simulink model "EKF_03"  (R2015a)
settings: Solver=ode45  StartTime=0.0  StopTime=40  RelTol=1e-3
model workspace: external: MAT-File Init_Model_02_Simulink.mat (data not in the file)
values from neighbouring files (symbols this model uses):
  Cov_nu = [0.005 0 0 0 ... (first row only)    [InitOOSM.m]    (also in InitSIL.m; Init_Model_02_Simulink.m; Init_Model_02_Simulink_SIL1.m)
  Cov_r = [0.003 0 0 ... (first row only)    [InitOOSM.m]    (also in InitSIL.m; Init_Model_02_Simulink.m; Init_Model_02_Simulink_SIL1.m)
  e_force_x = 0    [InitOOSM.m]    (also in InitSIL.m; Init_Model_02_Simulink.m; Init_Model_02_Simulink_SIL1.m)
  e_force_y = 0    [InitOOSM.m]    (also in InitSIL.m; Init_Model_02_Simulink.m; Init_Model_02_Simulink_SIL1.m)
  e_force_z = 0    [InitOOSM.m]    (also in InitSIL.m; Init_Model_02_Simulink.m; Init_Model_02_Simulink_SIL1.m)
  ita = [0.5;0.5;0.5;0.5]    [InitOOSM.m]    (also in InitSIL.m; Init_Model_02_Simulink.m = [0.12; 0.05; -0.15; 0.98]; Init_Model_02_Simulink_SIL1.m)
  n = 0.00    (= 0)    [InitOOSM.m]    (also in InitSIL.m; Init_Model_02_Simulink.m = 0.0012; Init_Model_02_Simulink_SIL1.m)
  P_d = Simulink.Signal    [InitOOSM.m]    (also in InitSIL.m; Init_Model_02_Simulink.m; Init_Model_02_Simulink_SIL1.m)
  P_k = Simulink.Signal    [InitOOSM.m]    (also in InitSIL.m; Init_Model_02_Simulink.m; Init_Model_02_Simulink_SIL1.m)
  p_x = 0.75    [InitOOSM.m]    (also in InitSIL.m; Init_Model_02_Simulink.m; Init_Model_02_Simulink_SIL1.m)
  p_y = 0.125    [InitOOSM.m]    (also in InitSIL.m; Init_Model_02_Simulink.m; Init_Model_02_Simulink_SIL1.m)
  p_z = -0.8    [InitOOSM.m]    (also in InitSIL.m; Init_Model_02_Simulink.m; Init_Model_02_Simulink_SIL1.m)
  parameter_gravitation = 3.986005E+14    (= 398600500000000)    [InitOOSM.m]    (also in InitSIL.m; Init_Model_02_Simulink.m; Init_Model_02_Simulink_SIL1.m)
  rho = [0.04;0;0.3]    [InitOOSM.m]    (also in InitSIL.m; Init_Model_02_Simulink.m = [0.2; 0.1; 0.05]; Init_Model_02_Simulink_SIL1.m)
  rho_c = [-0.00017;   -0.9780;   -0.1854]    [InitOOSM.m]    (also in InitSIL.m = [0.00036;   -0.9865;   -0.1854]; Init_Model_02_Simulink.m = [0; 0; 0.9]; Init_Model_02_Simulink_SIL1.m = [0.00036;   -0.9865;   -0.1854])
  sig_f = 2E-6    (= 2e-06)    [InitOOSM.m]    (also in InitSIL.m; Init_Model_02_Simulink.m; Init_Model_02_Simulink_SIL1.m)
  sig_tau = 2.5E-5    (= 2.5e-05)    [InitOOSM.m]    (also in InitSIL.m; Init_Model_02_Simulink.m; Init_Model_02_Simulink_SIL1.m)
  t_delta = 0.2    [InitOOSM.m]    (also in InitSIL.m; Init_Model_02_Simulink.m = 0.1; Init_Model_02_Simulink_SIL1.m)
  t_Kalman = 0.01    [InitOOSM.m]    (also in InitSIL.m; Init_Model_02_Simulink.m; Init_Model_02_Simulink_SIL1.m)
  t_Sim = 0.001    [InitOOSM.m]    (also in InitSIL.m; Init_Model_02_Simulink.m; Init_Model_02_Simulink_SIL1.m)
  tau_1 = 0    [InitOOSM.m]    (also in InitSIL.m; Init_Model_02_Simulink.m; Init_Model_02_Simulink_SIL1.m)
  tau_2 = 0    [InitOOSM.m]    (also in InitSIL.m; Init_Model_02_Simulink.m; Init_Model_02_Simulink_SIL1.m)
  tau_3 = 0    [InitOOSM.m]    (also in InitSIL.m; Init_Model_02_Simulink.m; Init_Model_02_Simulink_SIL1.m)
  U_n_d = Simulink.Signal    [InitOOSM.m]    (also in InitSIL.m; Init_Model_02_Simulink.m; Init_Model_02_Simulink_SIL1.m)
  X_a_0 = [0; 0; 0; 1; 0; 0; 0; 0; 0; 0; 0; 0; 0;0;0;0;0;0;0;1]    [InitOOSM.m]    (also in InitSIL.m = [0; 0; 0; 1; 0; 0; 0; 0; 0; 0; 0; 0; 0]; Init_Model_02_Simulink.m = [0; 0; 0; 1; 0; 0; 0; 0; 0; 0; 0; 0; 0]; Init_Model_02_Simulink_SIL1.m = [0;0;0.707;0.707;0.2;-0.02;0.0001;0.02;-1.80;0.50;-0.05;0.00)
  x_d = Simulink.Signal    [InitOOSM.m]    (also in InitSIL.m; Init_Model_02_Simulink.m; Init_Model_02_Simulink_SIL1.m)
  x_k = Simulink.Signal    [InitOOSM.m]    (also in InitSIL.m; Init_Model_02_Simulink.m; Init_Model_02_Simulink_SIL1.m)
undefined symbols (not defined in the file or in its folder): des, gcbh
libraries: simulink x5, dspmtrx3 x1
(part 3 of 5)

== system EKF_03/OOSM_KF/OOSM_KF/Initialize OOSM/Create State error covariance (P) ==
  X_a : Inport
  P_previous : Inport  Port=2
  del_t : Inport  Port=3
  Add : Sum
  Math Function : Math  Operator=transpose  SaturateOnIntegerOverflow=on
  Matrix Concatenate : Concatenate  Mode=Multidimensional array  ConcatenateDimension=2
  Matrix Concatenate1 : Concatenate  Mode=Multidimensional array
  Matrix Concatenate2 : Concatenate  Mode=Multidimensional array  ConcatenateDimension=2
  Process noise covariance [rotational] : Subsystem
  Process noise covariance [translational] : Subsystem
  Product : Product  Inputs=3  Multiplication=Matrix(*)
  State Propagation : Subsystem
  zeros(6,6) : Constant  Value=zeros(6,6)
  P_current : Outport
  wires:
  Math Function/1 -> Product/3
  P_previous/1 -> Product/2
  Add/1 -> P_current/1
  X_a/1 -> State Propagation/1("X_a(t)\t")
  Product/1 -> Add/2
  Matrix Concatenate1/1 -> Add/1
  Matrix Concatenate2/1 -> Matrix Concatenate1/2
  Matrix Concatenate/1 -> Matrix Concatenate1/1
  Process noise covariance [translational]/1(Q_t) -> Matrix Concatenate2/2
  zeros(6,6)/1 -> Matrix Concatenate2/1, Matrix Concatenate/2
  Process noise covariance [rotational]/1(Q_r) -> Matrix Concatenate/1
  State Propagation/1(Phi) -> Math Function/1, Product/1, Process noise covariance [rotational]/1(Phi)
  del_t/1 -> State Propagation/2(del_t), Process noise covariance [rotational]/2(del_t), Process noise covariance [translational]/1(del_t)

== system EKF_03/OOSM_KF/OOSM_KF/Initialize OOSM/Propagate_state (full) ==
  X_a(k-n) : Inport
  del_t : Inport  Port=2
  Bus Selector : BusSelector  OutputSignals=omega,r,r_dot
  Create q_nominal : Subsystem  TreatAsAtomicUnit=on
  Data Store Write : DataStoreWrite  DataStoreName=q_nominal_d
  Mux : Mux  Inputs=3
  Mux1 : Mux  Inputs=2
  Product : Product  Multiplication=Matrix(*)
  Selector : Selector  NumberOfDimensions=2  InputPortWidth=3  IndexOptions=Index vector (dialog),Index vector (dialog)  Indices=[4:12],[4:12]  OutputSizes=1,1
  State Propagation1 : Subsystem
  X_a(k-n,d) : Outport
  wires:
  X_a(k-n)/1 -> Bus Selector/1, Create q_nominal/1(X_a), State Propagation1/1("X_a(t)\t")
  Mux1/1 -> X_a(k-n,d)/1
  Bus Selector/1 -> Mux/1  "<omega>"
  Bus Selector/2 -> Mux/2  "<r>"
  Selector/1 -> Product/1
  Mux/1 -> Product/2
  Bus Selector/3 -> Mux/3  "<r_dot>"
  Product/1 -> Mux1/2
  Create q_nominal/1(Out1) -> Data Store Write/1, Mux1/1
  State Propagation1/1(Phi) -> Selector/1
  del_t/1 -> Create q_nominal/2(del_t), State Propagation1/2(del_t)

== system EKF_03/OOSM_KF/OOSM_KF/Initialize OOSM/State Propagation ==
  "X_a(t)\t" : Inport
  del_t : Inport  Port=2
  Create M : Subsystem
  MATLAB Function : MATLAB Function  TreatAsAtomicUnit=on
  n : Constant  Value=n
  p : Constant  Value=[p_x;p_y;p_z]
  Phi : Outport
  wires:
  p/1 -> Create M/2(p), MATLAB Function/4(p)
  n/1 -> MATLAB Function/2(n)
  del_t/1 -> MATLAB Function/3(t_Kalman)
  MATLAB Function/1(Phi) -> Phi/1
  "X_a(t)\t"/1 -> Create M/1("X_a "), MATLAB Function/1(X_a)
  Create M/1(M) -> MATLAB Function/5(M)

== system EKF_03/OOSM_KF/OOSM_KF/State Propagation1/Create M ==
  "X_a " : Inport
  p : Inport  Port=2
  0 : Constant  Value=0
  Bus Selector1 : BusSelector  OutputSignals=omega
  Bus Selector2 : BusSelector  OutputSignals=omega_x,omega_y,omega_z
  Create 3x3 matrix : Subsystem
  Demux : Demux  Outputs=3
  Product{,1..5} (6 alike) : Product
  M : Outport
  wires:
  Demux/1 -> Product1/1, Product/1
  p/1 -> Demux/1
  0/1 -> Create 3x3 matrix/1(a11), Create 3x3 matrix/9(a33), Create 3x3 matrix/5(a22)
  Product4/1 -> Create 3x3 matrix/7(a31)
  Product1/1 -> Create 3x3 matrix/3(a13)
  Bus Selector2/3 -> Product/2, Product2/2  "<omega_z>"
  Product5/1 -> Create 3x3 matrix/8(a32)
  Demux/3 -> Product5/1, Product4/1
  Bus Selector1/1 -> Bus Selector2/1  "<omega>"
  Product2/1 -> Create 3x3 matrix/4(a21)
  Demux/2 -> Product3/1, Product2/1
  Product/1 -> Create 3x3 matrix/2(a12)
  Bus Selector2/2 -> Product1/2, Product4/2  "<omega_y>"
  Create 3x3 matrix/1(Matrix) -> M/1
  Bus Selector2/1 -> Product5/2, Product3/2  "<omega_x>"
  Product3/1 -> Create 3x3 matrix/6(a23)
  "X_a "/1 -> Bus Selector1/1

== system EKF_03/OOSM_KF/Subsystem/Enabled Subsystem/Create H_k ==
  rho : Inport
  q_nominal : Inport  Port=2
  "Create Rotation Matrix " : Subsystem
  Create Skew Symmetric : Subsystem
  Gain : Gain  Gain=-2
  Matrix Concatenate : Concatenate  NumInputs=4  Mode=Multidimensional array  ConcatenateDimension=2
  Matrix Concatenate1 : Concatenate  NumInputs=4  Mode=Multidimensional array  ConcatenateDimension=2
  Matrix Concatenate2 : Concatenate  Mode=Multidimensional array
  Product : Product  Multiplication=Matrix(*)
  eye_3_3 : Constant  Value=eye(3,3)
  zeros_3_3 : Constant  Value=zeros(3,3)
  H_k : Outport
  wires:
  q_nominal/1 -> "Create Rotation Matrix "/1(q)
  Matrix Concatenate2/1 -> H_k/1
  "Create Rotation Matrix "/1(R) -> Product/1
  Product/1 -> Gain/1
  eye_3_3/1 -> Matrix Concatenate1/1, Matrix Concatenate/3
  zeros_3_3/1 -> Matrix Concatenate1/2, Matrix Concatenate1/4, Matrix Concatenate1/3, Matrix Concatenate/4, Matrix Concatenate/2
  Create Skew Symmetric/1(skew symmetric Matrix) -> Product/2
  Gain/1 -> Matrix Concatenate/1
  rho/1 -> Create Skew Symmetric/1(vector)
  Matrix Concatenate1/1 -> Matrix Concatenate2/2
  Matrix Concatenate/1 -> Matrix Concatenate2/1

== system EKF_03/Plant/Dynamic Model (Differential equations)/Orbital Dynamics /Create Skew Symmetric ==
  vector : Inport
  0 : Constant  Value=0
  Create 3x3 matrix : Subsystem
  Demux : Demux  Outputs=3
  Demux1 : Demux  Outputs=3
  Gain : Gain  Gain=-1
  skew symmetric Matrix : Outport
  wires:
  0/1 -> Create 3x3 matrix/1(a11), Create 3x3 matrix/5(a22), Create 3x3 matrix/9(a33)
  Demux/3 -> Create 3x3 matrix/2(a12)
  Demux1/2 -> Create 3x3 matrix/3(a13)
  Demux1/3 -> Create 3x3 matrix/4(a21)
  Demux/1 -> Create 3x3 matrix/6(a23)
  vector/1 -> Demux1/1, Gain/1
  Create 3x3 matrix/1(Matrix) -> skew symmetric Matrix/1
  Gain/1 -> Demux/1
  Demux/2 -> Create 3x3 matrix/7(a31)
  Demux1/1 -> Create 3x3 matrix/8(a32)

== system EKF_03/Plant/Dynamic Model (Differential equations)/Orbital Dynamics /norm  ==
  vector : Inport
  Dot Product : DotProduct  InputSameDT=on  OutDataTypeStr=Inherit: Inherit via internal rule
  Sqrt : Sqrt  SaturateOnIntegerOverflow=on
  "norm " : Outport
  wires:
  Dot Product/1 -> Sqrt/1
  vector/1 -> Dot Product/2, Dot Product/1
  Sqrt/1 -> "norm "/1

== system EKF_03/Plant/Dynamic Model (Differential equations)/Rotational Dynamics/Create  J ==
  p : Inport
  0 : Constant  Value=0
  1 : Constant
  Create 3x3 matrix : Subsystem
  Fcn : Fcn  Expr=1-u(2)/1+u(1)
  Fcn1 : Fcn  Expr=1+u(3)/1-u(1)
  "J_k " : Outport
  wires:
  Fcn/1 -> Create 3x3 matrix/5(a22)
  p/1 -> Fcn1/1, Fcn/1
  0/1 -> Create 3x3 matrix/2(a12), Create 3x3 matrix/3(a13), Create 3x3 matrix/4(a21), Create 3x3 matrix/6(a23), Create 3x3 matrix/7(a31), Create 3x3 matrix/8(a32)
  Create 3x3 matrix/1(Matrix) -> "J_k "/1
  Fcn1/1 -> Create 3x3 matrix/9(a33)
  1/1 -> Create 3x3 matrix/1(a11)

== system EKF_03/Plant/Dynamic Model (Differential equations)/Rotational Dynamics/Create Psi ==
  "omega " : Inport
  p : Inport  Port=2
  Create Psi : Concatenate  NumInputs=3
  Demux : Demux  Outputs=3
  Demux1 : Demux  Outputs=3
  Product{,1..5} (6 alike) : Product
  Psi : Outport
  wires:
  Demux1/3 -> Product1/2, Product3/2
  p/1 -> Demux/1
  Demux/3 -> Product4/1
  Product4/1 -> Create Psi/3
  Demux1/1 -> Product5/2, Product3/1
  Demux1/2 -> Product1/1, Product5/1
  Product2/1 -> Create Psi/2
  Demux/1 -> Product/1
  Create Psi/1 -> Psi/1
  Demux/2 -> Product2/1
  Product/1 -> Create Psi/1
  Product1/1 -> Product/2
  Product5/1 -> Product4/2
  Product3/1 -> Product2/2
  "omega "/1 -> Demux1/1

== system EKF_03/Plots and display/Create Measurements [Pose]1/Create Measurements [Position]/Create Rotation Matrix  ==
  q : Inport
  Add : Sum
  Add5 : Sum  Inputs=+++
  Constant1 : Constant  Value=-1
  Create Skew Symmetric : Subsystem
  Gain : Gain  Gain=2
  Gain1 : Gain  Gain=2
  Gain2 : Gain  Gain=2
  I : Constant  Value=eye(3,3)
  Math Function : Math  Operator=square  SaturateOnIntegerOverflow=on
  Math Function1 : Math  Operator=transpose  SaturateOnIntegerOverflow=on
  Product1 : Product
  Product2 : Product
  Product3 : Product  Multiplication=Matrix(*)
  Selector2 : Selector  NumberOfDimensions=2  InputPortWidth=3  IndexOptions=Index vector (dialog),Index vector (dialog)  Indices=[1 2 3],1  OutputSizes=1,1
  Selector3 : Selector  NumberOfDimensions=2  InputPortWidth=3  IndexOptions=Index vector (dialog),Index vector (dialog)  Indices=[4],1  OutputSizes=1,1
  R : Outport
  wires:
  q/1 -> Selector2/1, Selector3/1
  Add5/1 -> R/1
  Product3/1 -> Gain2/1
  Math Function1/1 -> Product3/2
  Product1/1 -> Add5/3
  Gain1/1 -> Product2/1
  Create Skew Symmetric/1(skew symmetric Matrix) -> Gain1/1
  Product2/1 -> Add5/2
  Gain2/1 -> Add5/1
  Selector2/1 -> Create Skew Symmetric/1(vector), Product3/1, Math Function1/1
  I/1 -> Product1/2
  Add/1 -> Product1/1
  Selector3/1 -> Math Function/1, Product2/2
  Constant1/1 -> Add/2
  Math Function/1 -> Gain/1
  Gain/1 -> Add/1

== system EKF_03/Create synthetic measurements [Pose]/Create Measurements [Position]/Create Rotation Matrix /Create Skew Symmetric/Create 3x3 matrix ==
  a11 : Inport
  a12 : Inport  Port=2
  a13 : Inport  Port=3
  a21 : Inport  Port=4
  a22 : Inport  Port=5
  a23 : Inport  Port=6
  a31 : Inport  Port=7
  a32 : Inport  Port=8
  a33 : Inport  Port=9
  Math Function : Math  Operator=transpose  SaturateOnIntegerOverflow=on
  Reshape (9) to [3x3] column-major : Reshape  OutputDimensionality=Customize  OutputDimensions=[3,3]
  Vector Concatenate : Concatenate  NumInputs=9
  Matrix : Outport
  wires:
  a33/1 -> Vector Concatenate/9
  a22/1 -> Vector Concatenate/5
  Vector Concatenate/1 -> Reshape (9) to [3x3] column-major/1
  a11/1 -> Vector Concatenate/1
  a12/1 -> Vector Concatenate/2
  a13/1 -> Vector Concatenate/3
  a23/1 -> Vector Concatenate/6
  a31/1 -> Vector Concatenate/7
  a32/1 -> Vector Concatenate/8
  a21/1 -> Vector Concatenate/4
  Reshape (9) to [3x3] column-major/1 -> Math Function/1
  Math Function/1 -> Matrix/1

== system EKF_03/EKF/Measurement Update/Compute_K_d/Create H_k/Create Rotation Matrix  ==
  q : Inport
  Add : Sum
  Add5 : Sum  Inputs=+++
  Constant1 : Constant  Value=-1
  Create Skew Symmetric : Subsystem
  Gain : Gain  Gain=2
  Gain1 : Gain  Gain=2
  Gain2 : Gain  Gain=2
  I : Constant  Value=eye(3,3)
  Math Function : Math  Operator=square  SaturateOnIntegerOverflow=on
  Math Function1 : Math  Operator=transpose  SaturateOnIntegerOverflow=on
  Product1 : Product
  Product2 : Product
  Product3 : Product  Multiplication=Matrix(*)
  Selector2 : Selector  NumberOfDimensions=2  InputPortWidth=3  IndexOptions=Index vector (dialog),Index vector (dialog)  Indices=[1 2 3],1  OutputSizes=1,1
  Selector3 : Selector  NumberOfDimensions=2  InputPortWidth=3  IndexOptions=Index vector (dialog),Index vector (dialog)  Indices=[4],1  OutputSizes=1,1
  R : Outport
  wires:
  Gain/1 -> Add/1
  Math Function/1 -> Gain/1
  Constant1/1 -> Add/2
  Selector3/1 -> Product2/2, Math Function/1
  Add/1 -> Product1/1
  I/1 -> Product1/2
  Selector2/1 -> Math Function1/1, Product3/1, Create Skew Symmetric/1(vector)
  Gain2/1 -> Add5/1
  Product2/1 -> Add5/2
  Create Skew Symmetric/1(skew symmetric Matrix) -> Gain1/1
  Gain1/1 -> Product2/1
  Product1/1 -> Add5/3
  Math Function1/1 -> Product3/2
  Product3/1 -> Gain2/1
  Add5/1 -> R/1
  q/1 -> Selector3/1, Selector2/1

== system EKF_03/EKF/Measurement Update/Compute_K_d/Create H_k/Create Skew Symmetric ==
  vector : Inport
  0 : Constant  Value=0
  Create 3x3 matrix : Subsystem
  Demux : Demux  Outputs=3
  Demux1 : Demux  Outputs=3
  Gain : Gain  Gain=-1
  skew symmetric Matrix : Outport
  wires:
  0/1 -> Create 3x3 matrix/1(a11), Create 3x3 matrix/9(a33), Create 3x3 matrix/5(a22)
  Demux/3 -> Create 3x3 matrix/2(a12)
  Demux1/2 -> Create 3x3 matrix/3(a13)
  Demux1/3 -> Create 3x3 matrix/4(a21)
  Demux/1 -> Create 3x3 matrix/6(a23)
  vector/1 -> Demux1/1, Gain/1
  Create 3x3 matrix/1(Matrix) -> skew symmetric Matrix/1
  Gain/1 -> Demux/1
  Demux/2 -> Create 3x3 matrix/7(a31)
  Demux1/1 -> Create 3x3 matrix/8(a32)

== system EKF_03/EKF/Measurement Update/Create H_k/Create Rotation Matrix /Create Skew Symmetric ==
  vector : Inport
  0 : Constant  Value=0
  Create 3x3 matrix : Subsystem
  Demux : Demux  Outputs=3
  Demux1 : Demux  Outputs=3
  Gain : Gain  Gain=-1
  skew symmetric Matrix : Outport
  wires:
  0/1 -> Create 3x3 matrix/1(a11), Create 3x3 matrix/9(a33), Create 3x3 matrix/5(a22)
  Demux/3 -> Create 3x3 matrix/2(a12)
  Demux1/2 -> Create 3x3 matrix/3(a13)
  Demux1/3 -> Create 3x3 matrix/4(a21)
  Demux/1 -> Create 3x3 matrix/6(a23)
  vector/1 -> Demux1/1, Gain/1
  Create 3x3 matrix/1(Matrix) -> skew symmetric Matrix/1
  Gain/1 -> Demux/1
  Demux/2 -> Create 3x3 matrix/7(a31)
  Demux1/1 -> Create 3x3 matrix/8(a32)

== system EKF_03/EKF/Measurement Update/Create H_k/Create Skew Symmetric/Create 3x3 matrix ==
  a11 : Inport
  a12 : Inport  Port=2
  a13 : Inport  Port=3
  a21 : Inport  Port=4
  a22 : Inport  Port=5
  a23 : Inport  Port=6
  a31 : Inport  Port=7
  a32 : Inport  Port=8
  a33 : Inport  Port=9
  Math Function : Math  Operator=transpose  SaturateOnIntegerOverflow=on
  Reshape (9) to [3x3] column-major : Reshape  OutputDimensionality=Customize  OutputDimensions=[3,3]
  Vector Concatenate : Concatenate  NumInputs=9
  Matrix : Outport
  wires:
  a33/1 -> Vector Concatenate/9
  a22/1 -> Vector Concatenate/5
  Vector Concatenate/1 -> Reshape (9) to [3x3] column-major/1
  a11/1 -> Vector Concatenate/1
  a12/1 -> Vector Concatenate/2
  a13/1 -> Vector Concatenate/3
  a23/1 -> Vector Concatenate/6
  a31/1 -> Vector Concatenate/7
  a32/1 -> Vector Concatenate/8
  a21/1 -> Vector Concatenate/4
  Reshape (9) to [3x3] column-major/1 -> Math Function/1
  Math Function/1 -> Matrix/1

== system EKF_03/EKF/Measurement Update/Create X_a from X/Create q_nominal /norm  ==
  vector : Inport
  Dot Product : DotProduct  InputSameDT=on  OutDataTypeStr=Inherit: Inherit via internal rule
  "norm " : Outport
  wires:
  vector/1 -> Dot Product/2, Dot Product/1
  Dot Product/1 -> "norm "/1

== system EKF_03/EKF/Measurement Update/Create h/Create Rotation Matrix /Create Skew Symmetric ==
  vector : Inport
  0 : Constant  Value=0
  Create 3x3 matrix : Subsystem
  Demux : Demux  Outputs=3
  Demux1 : Demux  Outputs=3
  Gain : Gain  Gain=-1
  skew symmetric Matrix : Outport
  wires:
  0/1 -> Create 3x3 matrix/1(a11), Create 3x3 matrix/9(a33), Create 3x3 matrix/5(a22)
  Demux/3 -> Create 3x3 matrix/2(a12)
  Demux1/2 -> Create 3x3 matrix/3(a13)
  Demux1/3 -> Create 3x3 matrix/4(a21)
  Demux/1 -> Create 3x3 matrix/6(a23)
  vector/1 -> Demux1/1, Gain/1
  Create 3x3 matrix/1(Matrix) -> skew symmetric Matrix/1
  Gain/1 -> Demux/1
  Demux/2 -> Create 3x3 matrix/7(a31)
  Demux1/1 -> Create 3x3 matrix/8(a32)

== system EKF_03/EKF/Measurement Update/Create h/Subsystem/norm  ==
  vector : Inport
  Dot Product : DotProduct  InputSameDT=on  OutDataTypeStr=Inherit: Inherit via internal rule
  "norm " : Outport
  wires:
  vector/1 -> Dot Product/2, Dot Product/1
  Dot Product/1 -> "norm "/1

== system EKF_03/EKF/Measurement Update/Create h_d/Create Rotation Matrix /Create Skew Symmetric ==
  vector : Inport
  0 : Constant  Value=0
  Create 3x3 matrix : Subsystem
  Demux : Demux  Outputs=3
  Demux1 : Demux  Outputs=3
  Gain : Gain  Gain=-1
  skew symmetric Matrix : Outport
  wires:
  Demux1/1 -> Create 3x3 matrix/8(a32)
  Demux/2 -> Create 3x3 matrix/7(a31)
  Gain/1 -> Demux/1
  Create 3x3 matrix/1(Matrix) -> skew symmetric Matrix/1
  vector/1 -> Gain/1, Demux1/1
  Demux/1 -> Create 3x3 matrix/6(a23)
  Demux1/3 -> Create 3x3 matrix/4(a21)
  Demux1/2 -> Create 3x3 matrix/3(a13)
  Demux/3 -> Create 3x3 matrix/2(a12)
  0/1 -> Create 3x3 matrix/5(a22), Create 3x3 matrix/9(a33), Create 3x3 matrix/1(a11)

== system EKF_03/EKF/Measurement Update/Create h_d/Subsystem/norm  ==
  vector : Inport
  Dot Product : DotProduct  InputSameDT=on  OutDataTypeStr=Inherit: Inherit via internal rule
  "norm " : Outport
  wires:
  Dot Product/1 -> "norm "/1
  vector/1 -> Dot Product/1, Dot Product/2

== system EKF_03/EKF/Measurement Update/Propagate_state (full)/Create q_nominal/Create Bus [State Vector,X_a]3 ==
  X : Inport
  Bus Creator2 : BusCreator
  Bus Creator3 : BusCreator  Inputs=3
  Bus Creator4 : BusCreator  Inputs=3
  Bus Creator5 : BusCreator  Inputs=3
  Bus Creator6 : BusCreator
  Demux1 : Demux  Outputs=13
  X_bus : Outport
  wires:
  Bus Creator2/1 -> Bus Creator6/1  "q_est"
  Bus Creator3/1 -> Bus Creator6/2  "omega"
  Bus Creator4/1 -> Bus Creator6/3  "r"
  Bus Creator5/1 -> Bus Creator6/4  "r_dot"
  Bus Creator6/1 -> X_bus/1
  X/1 -> Demux1/1
  Demux1/1 -> Bus Creator2/1  "q_est_1"
  Demux1/2 -> Bus Creator2/2  "q_est_2"
  Demux1/3 -> Bus Creator2/3  "q_est_3"
  Demux1/4 -> Bus Creator2/4  "q_est_0"
  Demux1/5 -> Bus Creator3/1  "omega_x"
  Demux1/6 -> Bus Creator3/2  "omega_y"
  Demux1/7 -> Bus Creator3/3  "omega_z"
  Demux1/8 -> Bus Creator4/1  "r_x"
  Demux1/9 -> Bus Creator4/2  "r_y"
  Demux1/10 -> Bus Creator4/3  "r_z"
  Demux1/11 -> Bus Creator5/1  "r_x_dot"
  Demux1/12 -> Bus Creator5/2  "r_y_dot"
  Demux1/13 -> Bus Creator5/3  "r_z_dot"

== system EKF_03/EKF/Measurement Update/Propagate_state (full)/Create q_nominal/Create nominal q ==
  q : Inport
  omega : Inport  Port=2
  del_t : Inport  Port=3
  Constant : Constant  Value=[0]
  Display : Display
  Display1 : Display
  Gain : Gain  Gain=0.5
  MATLAB Function : MATLAB Function  TreatAsAtomicUnit=on
  MATLAB Function1 : MATLAB Function  TreatAsAtomicUnit=on
  Product : Product
  Product1 : Product  Multiplication=Matrix(*)
  Vector Concatenate : Concatenate
  flag : Constant  Value=0
  q_nominal : Outport
  wires:
  MATLAB Function/1(CrossTensor) -> Product/1
  del_t/1 -> Product/2
  Gain/1 -> MATLAB Function1/1(A)
  omega/1 -> Vector Concatenate/1
  Constant/1 -> Vector Concatenate/2
  flag/1 -> MATLAB Function/2(flag)
  Product/1 -> Gain/1
  Vector Concatenate/1 -> MATLAB Function/1(q)
  MATLAB Function1/1(exponent_A) -> Product1/1
  Product1/1 -> Display/1, q_nominal/1
  q/1 -> Display1/1, Product1/2

== system EKF_03/EKF/Measurement Update/Propagate_state (full)/State Propagation1/Create M ==
  "X_a " : Inport
  p : Inport  Port=2
  0 : Constant  Value=0
  Bus Selector1 : BusSelector  OutputSignals=omega
  Bus Selector2 : BusSelector  OutputSignals=omega_x,omega_y,omega_z
  Create 3x3 matrix : Subsystem
  Demux : Demux  Outputs=3
  Product{,1..5} (6 alike) : Product
  M : Outport
  wires:
  Demux/1 -> Product1/1, Product/1
  p/1 -> Demux/1
  0/1 -> Create 3x3 matrix/1(a11), Create 3x3 matrix/9(a33), Create 3x3 matrix/5(a22)
  Product4/1 -> Create 3x3 matrix/7(a31)
  Product1/1 -> Create 3x3 matrix/3(a13)
  Bus Selector2/3 -> Product/2, Product2/2  "<omega_z>"
  Product5/1 -> Create 3x3 matrix/8(a32)
  Demux/3 -> Product5/1, Product4/1
  Bus Selector1/1 -> Bus Selector2/1  "<omega>"
  Product2/1 -> Create 3x3 matrix/4(a21)
  Demux/2 -> Product3/1, Product2/1
  Product/1 -> Create 3x3 matrix/2(a12)
  Bus Selector2/2 -> Product1/2, Product4/2  "<omega_y>"
  Create 3x3 matrix/1(Matrix) -> M/1
  Bus Selector2/1 -> Product5/2, Product3/2  "<omega_x>"
  Product3/1 -> Create 3x3 matrix/6(a23)
  "X_a "/1 -> Bus Selector1/1

== system EKF_03/EKF/Predictor/Create State error covariance (P)/State Propagation/Create M ==
  "X_a " : Inport
  p : Inport  Port=2
  0 : Constant  Value=0
  Bus Selector1 : BusSelector  OutputSignals=omega
  Bus Selector2 : BusSelector  OutputSignals=omega_x,omega_y,omega_z
  Create 3x3 matrix : Subsystem
  Demux : Demux  Outputs=3
  Product{,1..5} (6 alike) : Product
  M : Outport
  wires:
  Demux/1 -> Product1/1, Product/1
  p/1 -> Demux/1
  0/1 -> Create 3x3 matrix/1(a11), Create 3x3 matrix/9(a33), Create 3x3 matrix/5(a22)
  Product4/1 -> Create 3x3 matrix/7(a31)
  Product1/1 -> Create 3x3 matrix/3(a13)
  Bus Selector2/3 -> Product/2, Product2/2  "<omega_z>"
  Product5/1 -> Create 3x3 matrix/8(a32)
  Demux/3 -> Product5/1, Product4/1
  Bus Selector1/1 -> Bus Selector2/1  "<omega>"
  Product2/1 -> Create 3x3 matrix/4(a21)
  Demux/2 -> Product3/1, Product2/1
  Product/1 -> Create 3x3 matrix/2(a12)
  Bus Selector2/2 -> Product1/2, Product4/2  "<omega_y>"
  Create 3x3 matrix/1(Matrix) -> M/1
  Bus Selector2/1 -> Product5/2, Product3/2  "<omega_x>"
  Product3/1 -> Create 3x3 matrix/6(a23)
  "X_a "/1 -> Bus Selector1/1

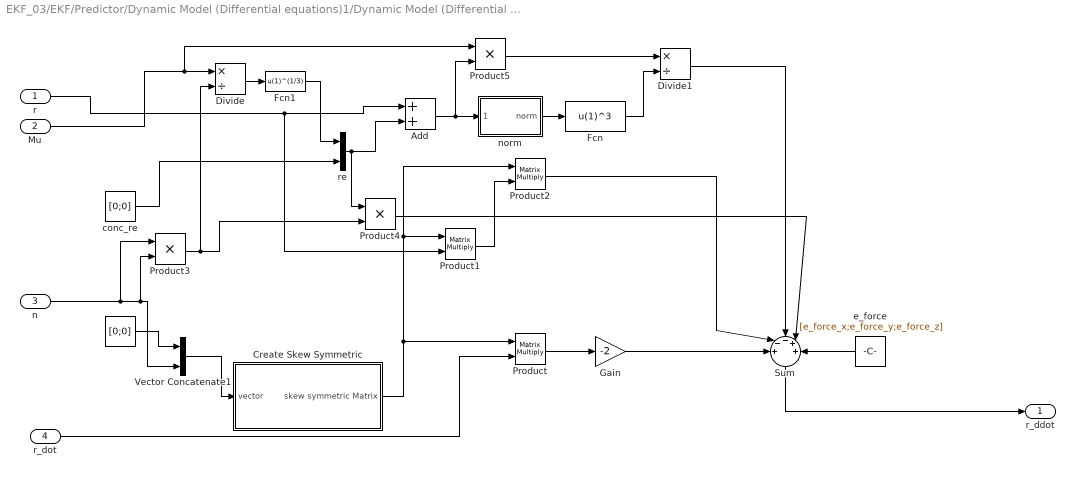
== system EKF_03/EKF/Predictor/Dynamic Model (Differential equations)1/Dynamic Model (Differential equations)/Orbital Dynamics  ==
  r : Inport
  Mu : Inport  Port=2
  n : Inport  Port=3
  "r_dot " : Inport  Port=4
  " " : Constant  Value=[0;0]  SampleTime=-1
  Add : Sum
  Create Skew Symmetric : Subsystem
  Divide : Product  Inputs=*/
  Divide1 : Product  Inputs=*/
  Fcn : Fcn  Expr=u(1)^3
  Fcn1 : Fcn  Expr=u(1)^(1/3)
  Gain : Gain  Gain=-2
  Product : Product  Multiplication=Matrix(*)
  Product1 : Product  Multiplication=Matrix(*)
  Product2 : Product  Multiplication=Matrix(*)
  Product3 : Product
  Product4 : Product
  Product5 : Product
  Sum : Sum  Inputs=+--++
  Vector Concatenate1 : Concatenate
  "conc_re " : Constant  Value=[0;0]  SampleTime=-1
  "e_force " : Constant  Value=[e_force_x;e_force_y;e_force_z]  SampleTime=-1
  "norm " : Subsystem
  re : Concatenate
  "r_ddot " : Outport
  wires:
  " "/1 -> Vector Concatenate1/1
  Create Skew Symmetric/1(skew symmetric Matrix) -> Product/1, Product1/1, Product2/1
  Product1/1 -> Product2/2
  Mu/1 -> Product5/1, Divide/1
  Product/1 -> Gain/1
  "conc_re "/1 -> re/2
  re/1 -> Product4/1, Add/2
  Product5/1 -> Divide1/1
  "norm "/1("norm ") -> Fcn/1
  n/1 -> Product3/2, Vector Concatenate1/2, Product3/1
  Product3/1 -> Divide/2, Product4/2
  Vector Concatenate1/1 -> Create Skew Symmetric/1(vector)
  Add/1 -> "norm "/1(vector), Product5/2
  Gain/1 -> Sum/1
  Product2/1 -> Sum/2
  r/1 -> Product1/2, Add/1
  Product4/1 -> Sum/4
  "r_dot "/1 -> Product/2
  Divide1/1 -> Sum/3
  Fcn1/1 -> re/1
  Fcn/1 -> Divide1/2
  Divide/1 -> Fcn1/1
  "e_force "/1 -> Sum/5
  Sum/1 -> "r_ddot "/1

== system EKF_03/EKF/Predictor/Dynamic Model (Differential equations)1/Dynamic Model (Differential equations)/Quaternion Kinematics ==
  q : Inport
  omega_rel : Inport  Port=2
  Constant2 : Constant  Value=0.5  SampleTime=-1
  MATLAB Function : MATLAB Function  TreatAsAtomicUnit=on
  Product : Product  Multiplication=Matrix(*)
  Product1 : Product
  flag : Constant  SampleTime=-1
  q_dot : Outport
  wires:
  MATLAB Function/1(CrossTensor) -> Product/1
  flag/1 -> MATLAB Function/2(flag)
  Constant2/1 -> Product1/2
  q/1 -> MATLAB Function/1(q)
  omega_rel/1 -> Product/2
  Product1/1 -> q_dot/1
  Product/1 -> Product1/1

== system EKF_03/EKF/Predictor/Dynamic Model (Differential equations)1/Dynamic Model (Differential equations)/Rotational Dynamics ==
  omega : Inport
  p : Inport  Port=2
  Add : Sum
  Create  J : Subsystem
  Create Psi : Subsystem
  Product : Product  Multiplication=Matrix(*)
  tau : Constant  Value=[tau_1;tau_2;tau_3]  SampleTime=-1
  omega_dot : Outport
  wires:
  omega/1 -> Create Psi/1("omega ")
  Create Psi/1(Psi) -> Add/1
  Add/1 -> omega_dot/1
  Product/1 -> Add/2
  p/1 -> Create Psi/2(p), Create  J/1(p)
  Create  J/1("J_k ") -> Product/1
  tau/1 -> Product/2

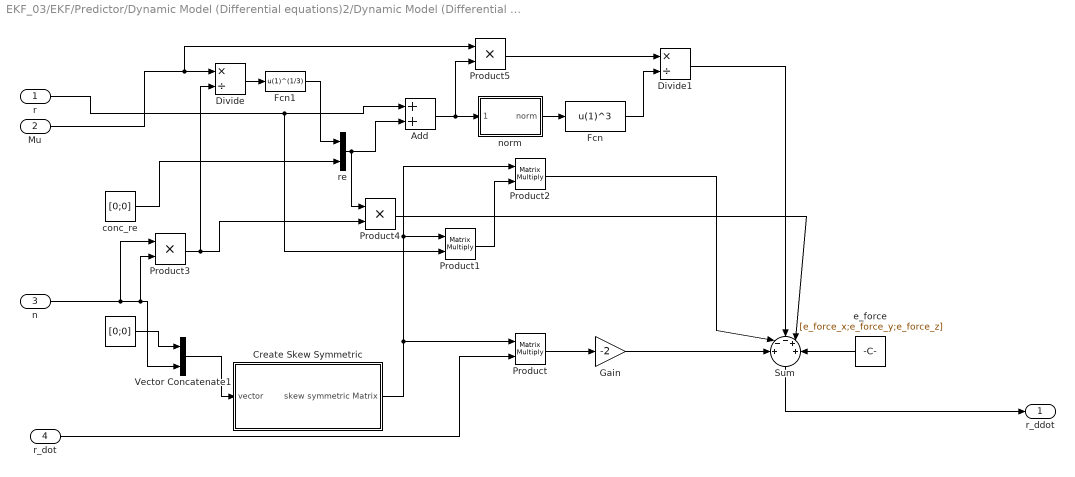
== system EKF_03/EKF/Predictor/Dynamic Model (Differential equations)2/Dynamic Model (Differential equations)/Orbital Dynamics  ==
  r : Inport
  Mu : Inport  Port=2
  n : Inport  Port=3
  "r_dot " : Inport  Port=4
  " " : Constant  Value=[0;0]  SampleTime=-1
  Add : Sum
  Create Skew Symmetric : Subsystem
  Divide : Product  Inputs=*/
  Divide1 : Product  Inputs=*/
  Fcn : Fcn  Expr=u(1)^3
  Fcn1 : Fcn  Expr=u(1)^(1/3)
  Gain : Gain  Gain=-2
  Product : Product  Multiplication=Matrix(*)
  Product1 : Product  Multiplication=Matrix(*)
  Product2 : Product  Multiplication=Matrix(*)
  Product3 : Product
  Product4 : Product
  Product5 : Product
  Sum : Sum  Inputs=+--++
  Vector Concatenate1 : Concatenate
  "conc_re " : Constant  Value=[0;0]  SampleTime=-1
  "e_force " : Constant  Value=[e_force_x;e_force_y;e_force_z]  SampleTime=-1
  "norm " : Subsystem
  re : Concatenate
  "r_ddot " : Outport
  wires:
  Sum/1 -> "r_ddot "/1
  "e_force "/1 -> Sum/5
  Divide/1 -> Fcn1/1
  Fcn/1 -> Divide1/2
  Fcn1/1 -> re/1
  Divide1/1 -> Sum/3
  "r_dot "/1 -> Product/2
  Product4/1 -> Sum/4
  r/1 -> Add/1, Product1/2
  Product2/1 -> Sum/2
  Gain/1 -> Sum/1
  Add/1 -> Product5/2, "norm "/1(vector)
  Vector Concatenate1/1 -> Create Skew Symmetric/1(vector)
  Product3/1 -> Product4/2, Divide/2
  n/1 -> Product3/1, Vector Concatenate1/2, Product3/2
  "norm "/1("norm ") -> Fcn/1
  Product5/1 -> Divide1/1
  re/1 -> Add/2, Product4/1
  "conc_re "/1 -> re/2
  Product/1 -> Gain/1
  Mu/1 -> Divide/1, Product5/1
  Product1/1 -> Product2/2
  Create Skew Symmetric/1(skew symmetric Matrix) -> Product2/1, Product1/1, Product/1
  " "/1 -> Vector Concatenate1/1

== system EKF_03/EKF/Predictor/Dynamic Model (Differential equations)2/Dynamic Model (Differential equations)/Quaternion Kinematics ==
  q : Inport
  omega_rel : Inport  Port=2
  Constant2 : Constant  Value=0.5  SampleTime=-1
  MATLAB Function : MATLAB Function  TreatAsAtomicUnit=on
  Product : Product  Multiplication=Matrix(*)
  Product1 : Product
  flag : Constant  SampleTime=-1
  q_dot : Outport
  wires:
  Product/1 -> Product1/1
  Product1/1 -> q_dot/1
  omega_rel/1 -> Product/2
  q/1 -> MATLAB Function/1(q)
  Constant2/1 -> Product1/2
  flag/1 -> MATLAB Function/2(flag)
  MATLAB Function/1(CrossTensor) -> Product/1

== system EKF_03/EKF/Predictor/Dynamic Model (Differential equations)2/Dynamic Model (Differential equations)/Rotational Dynamics ==
  omega : Inport
  p : Inport  Port=2
  Add : Sum
  Create  J : Subsystem
  Create Psi : Subsystem
  Product : Product  Multiplication=Matrix(*)
  tau : Constant  Value=[tau_1;tau_2;tau_3]  SampleTime=-1
  omega_dot : Outport
  wires:
  tau/1 -> Product/2
  Create  J/1("J_k ") -> Product/1
  p/1 -> Create  J/1(p), Create Psi/2(p)
  Product/1 -> Add/2
  Add/1 -> omega_dot/1
  Create Psi/1(Psi) -> Add/1
  omega/1 -> Create Psi/1("omega ")

== system EKF_03/OOSM_KF/OOSM_KF/Initialize OOSM/Create State error covariance (P)/Process noise covariance [rotational] ==
  Phi : Inport
  del_t : Inport  Port=2
  Process Noise covariance : MATLAB Function  TreatAsAtomicUnit=on
  p : Constant  Value=[p_x;p_y;p_z]
  sig_tau : Constant  Value=sig_tau
  Q_r : Outport
  wires:
  Phi/1 -> Process Noise covariance/1(Phi)
  del_t/1 -> Process Noise covariance/3(t_delta)
  sig_tau/1 -> Process Noise covariance/4(tau)
  p/1 -> Process Noise covariance/6(p)
  Process Noise covariance/1(Q_r) -> Q_r/1

== system EKF_03/OOSM_KF/OOSM_KF/Initialize OOSM/Create State error covariance (P)/Process noise covariance [translational] ==
  del_t : Inport
  Process noise covariance [translational] : MATLAB Function  TreatAsAtomicUnit=on
  n : Constant  Value=n
  sig_f : Constant  Value=sig_f
  Q_t : Outport
  wires:
  n/1 -> Process noise covariance [translational]/2(n)
  del_t/1 -> Process noise covariance [translational]/1(t_Kalman)
  sig_f/1 -> Process noise covariance [translational]/3(sigma_f)
  Process noise covariance [translational]/1(Q_t_k) -> Q_t/1

== system EKF_03/OOSM_KF/OOSM_KF/Initialize OOSM/Create State error covariance (P)/State Propagation ==
  "X_a(t)\t" : Inport
  del_t : Inport  Port=2
  Create M : Subsystem
  MATLAB Function : MATLAB Function  TreatAsAtomicUnit=on
  n : Constant  Value=n
  p : Constant  Value=[p_x;p_y;p_z]
  Phi : Outport
  wires:
  p/1 -> Create M/2(p), MATLAB Function/4(p)
  n/1 -> MATLAB Function/2(n)
  del_t/1 -> MATLAB Function/3(t_Kalman)
  MATLAB Function/1(Phi) -> Phi/1
  "X_a(t)\t"/1 -> Create M/1("X_a "), MATLAB Function/1(X_a)
  Create M/1(M) -> MATLAB Function/5(M)

== system EKF_03/OOSM_KF/OOSM_KF/Initialize OOSM/Propagate_state (full)/Create q_nominal ==
  X_a : Inport
  del_t : Inport  Port=2
  Bus Selector1 : BusSelector  OutputSignals=q_est,omega
  Create Bus [State Vector,X_a]3 : Subsystem
  Create nominal q : Subsystem
  Scope6 : Scope
      settings: ShowLegends=on  SaveName=ScopeData21
  Out1 : Outport
  wires:
  Bus Selector1/2 -> Create nominal q/2(omega)  "<omega>"
  Create nominal q/1(q_nominal) -> Scope6/1, Out1/1
  Bus Selector1/1 -> Create nominal q/1(q)  "<q_est>"
  Create Bus [State Vector,X_a]3/1(X_bus) -> Bus Selector1/1
  X_a/1 -> Create Bus [State Vector,X_a]3/1(X)
  del_t/1 -> Create nominal q/3(del_t)

== system EKF_03/OOSM_KF/OOSM_KF/Initialize OOSM/Propagate_state (full)/State Propagation1 ==
  "X_a(t)\t" : Inport
  del_t : Inport  Port=2
  Create M : Subsystem
  MATLAB Function : MATLAB Function  TreatAsAtomicUnit=on
  n : Constant  Value=n
  p : Constant  Value=[p_x;p_y;p_z]
  Phi : Outport
  wires:
  p/1 -> Create M/2(p), MATLAB Function/4(p)
  n/1 -> MATLAB Function/2(n)
  del_t/1 -> MATLAB Function/3(t_Kalman)
  MATLAB Function/1(Phi) -> Phi/1
  "X_a(t)\t"/1 -> Create M/1("X_a "), MATLAB Function/1(X_a)
  Create M/1(M) -> MATLAB Function/5(M)

== system EKF_03/OOSM_KF/OOSM_KF/Initialize OOSM/State Propagation/Create M ==
  "X_a " : Inport
  p : Inport  Port=2
  0 : Constant  Value=0
  Bus Selector1 : BusSelector  OutputSignals=omega
  Bus Selector2 : BusSelector  OutputSignals=omega_x,omega_y,omega_z
  Create 3x3 matrix : Subsystem
  Demux : Demux  Outputs=3
  Product{,1..5} (6 alike) : Product
  M : Outport
  wires:
  Demux/1 -> Product1/1, Product/1
  p/1 -> Demux/1
  0/1 -> Create 3x3 matrix/1(a11), Create 3x3 matrix/9(a33), Create 3x3 matrix/5(a22)
  Product4/1 -> Create 3x3 matrix/7(a31)
  Product1/1 -> Create 3x3 matrix/3(a13)
  Bus Selector2/3 -> Product/2, Product2/2  "<omega_z>"
  Product5/1 -> Create 3x3 matrix/8(a32)
  Demux/3 -> Product5/1, Product4/1
  Bus Selector1/1 -> Bus Selector2/1  "<omega>"
  Product2/1 -> Create 3x3 matrix/4(a21)
  Demux/2 -> Product3/1, Product2/1
  Product/1 -> Create 3x3 matrix/2(a12)
  Bus Selector2/2 -> Product1/2, Product4/2  "<omega_y>"
  Create 3x3 matrix/1(Matrix) -> M/1
  Bus Selector2/1 -> Product5/2, Product3/2  "<omega_x>"
  Product3/1 -> Create 3x3 matrix/6(a23)
  "X_a "/1 -> Bus Selector1/1

== system EKF_03/OOSM_KF/OOSM_KF/State Propagation1/Create M/Create 3x3 matrix ==
  a11 : Inport
  a12 : Inport  Port=2
  a13 : Inport  Port=3
  a21 : Inport  Port=4
  a22 : Inport  Port=5
  a23 : Inport  Port=6
  a31 : Inport  Port=7
  a32 : Inport  Port=8
  a33 : Inport  Port=9
  Math Function : Math  Operator=transpose  SaturateOnIntegerOverflow=on
  Reshape (9) to [3x3] column-major : Reshape  OutputDimensionality=Customize  OutputDimensions=[3,3]
  Vector Concatenate : Concatenate  NumInputs=9
  Matrix : Outport
  wires:
  a33/1 -> Vector Concatenate/9
  a22/1 -> Vector Concatenate/5
  Vector Concatenate/1 -> Reshape (9) to [3x3] column-major/1
  a11/1 -> Vector Concatenate/1
  a12/1 -> Vector Concatenate/2
  a13/1 -> Vector Concatenate/3
  a23/1 -> Vector Concatenate/6
  a31/1 -> Vector Concatenate/7
  a32/1 -> Vector Concatenate/8
  a21/1 -> Vector Concatenate/4
  Reshape (9) to [3x3] column-major/1 -> Math Function/1
  Math Function/1 -> Matrix/1

== system EKF_03/OOSM_KF/Subsystem/Enabled Subsystem/Create H_k/Create Rotation Matrix  ==
  q : Inport
  Add : Sum
  Add5 : Sum  Inputs=+++
  Constant1 : Constant  Value=-1
  Create Skew Symmetric : Subsystem
  Gain : Gain  Gain=2
  Gain1 : Gain  Gain=2
  Gain2 : Gain  Gain=2
  I : Constant  Value=eye(3,3)
  Math Function : Math  Operator=square  SaturateOnIntegerOverflow=on
  Math Function1 : Math  Operator=transpose  SaturateOnIntegerOverflow=on
  Product1 : Product
  Product2 : Product
  Product3 : Product  Multiplication=Matrix(*)
  Selector2 : Selector  NumberOfDimensions=2  InputPortWidth=3  IndexOptions=Index vector (dialog),Index vector (dialog)  Indices=[1 2 3],1  OutputSizes=1,1
  Selector3 : Selector  NumberOfDimensions=2  InputPortWidth=3  IndexOptions=Index vector (dialog),Index vector (dialog)  Indices=[4],1  OutputSizes=1,1
  R : Outport
  wires:
  Gain/1 -> Add/1
  Math Function/1 -> Gain/1
  Constant1/1 -> Add/2
  Selector3/1 -> Product2/2, Math Function/1
  Add/1 -> Product1/1
  I/1 -> Product1/2
  Selector2/1 -> Math Function1/1, Product3/1, Create Skew Symmetric/1(vector)
  Gain2/1 -> Add5/1
  Product2/1 -> Add5/2
  Create Skew Symmetric/1(skew symmetric Matrix) -> Gain1/1
  Gain1/1 -> Product2/1
  Product1/1 -> Add5/3
  Math Function1/1 -> Product3/2
  Product3/1 -> Gain2/1
  Add5/1 -> R/1
  q/1 -> Selector3/1, Selector2/1

== system EKF_03/OOSM_KF/Subsystem/Enabled Subsystem/Create H_k/Create Skew Symmetric ==
  vector : Inport
  0 : Constant  Value=0
  Create 3x3 matrix : Subsystem
  Demux : Demux  Outputs=3
  Demux1 : Demux  Outputs=3
  Gain : Gain  Gain=-1
  skew symmetric Matrix : Outport
  wires:
  0/1 -> Create 3x3 matrix/1(a11), Create 3x3 matrix/9(a33), Create 3x3 matrix/5(a22)
  Demux/3 -> Create 3x3 matrix/2(a12)
  Demux1/2 -> Create 3x3 matrix/3(a13)
  Demux1/3 -> Create 3x3 matrix/4(a21)
  Demux/1 -> Create 3x3 matrix/6(a23)
  vector/1 -> Demux1/1, Gain/1
  Create 3x3 matrix/1(Matrix) -> skew symmetric Matrix/1
  Gain/1 -> Demux/1
  Demux/2 -> Create 3x3 matrix/7(a31)
  Demux1/1 -> Create 3x3 matrix/8(a32)

== system EKF_03/Plant/Dynamic Model (Differential equations)/Orbital Dynamics /Create Skew Symmetric/Create 3x3 matrix ==
  a11 : Inport
  a12 : Inport  Port=2
  a13 : Inport  Port=3
  a21 : Inport  Port=4
  a22 : Inport  Port=5
  a23 : Inport  Port=6
  a31 : Inport  Port=7
  a32 : Inport  Port=8
  a33 : Inport  Port=9
  Math Function : Math  Operator=transpose  SaturateOnIntegerOverflow=on
  Reshape (9) to [3x3] column-major : Reshape  OutputDimensionality=Customize  OutputDimensions=[3,3]
  Vector Concatenate : Concatenate  NumInputs=9
  Matrix : Outport
  wires:
  a33/1 -> Vector Concatenate/9
  a22/1 -> Vector Concatenate/5
  Vector Concatenate/1 -> Reshape (9) to [3x3] column-major/1
  a11/1 -> Vector Concatenate/1
  a12/1 -> Vector Concatenate/2
  a13/1 -> Vector Concatenate/3
  a23/1 -> Vector Concatenate/6
  a31/1 -> Vector Concatenate/7
  a32/1 -> Vector Concatenate/8
  a21/1 -> Vector Concatenate/4
  Reshape (9) to [3x3] column-major/1 -> Math Function/1
  Math Function/1 -> Matrix/1

== system EKF_03/Plant/Dynamic Model (Differential equations)/Rotational Dynamics/Create  J/Create 3x3 matrix ==
  a11 : Inport
  a12 : Inport  Port=2
  a13 : Inport  Port=3
  a21 : Inport  Port=4
  a22 : Inport  Port=5
  a23 : Inport  Port=6
  a31 : Inport  Port=7
  a32 : Inport  Port=8
  a33 : Inport  Port=9
  Math Function : Math  Operator=transpose  SaturateOnIntegerOverflow=on
  Reshape (9) to [3x3] column-major : Reshape  OutputDimensionality=Customize  OutputDimensions=[3,3]
  Vector Concatenate : Concatenate  NumInputs=9
  Matrix : Outport
  wires:
  a33/1 -> Vector Concatenate/9
  a22/1 -> Vector Concatenate/5
  Vector Concatenate/1 -> Reshape (9) to [3x3] column-major/1
  a11/1 -> Vector Concatenate/1
  a12/1 -> Vector Concatenate/2
  a13/1 -> Vector Concatenate/3
  a23/1 -> Vector Concatenate/6
  a31/1 -> Vector Concatenate/7
  a32/1 -> Vector Concatenate/8
  a21/1 -> Vector Concatenate/4
  Reshape (9) to [3x3] column-major/1 -> Math Function/1
  Math Function/1 -> Matrix/1

== system EKF_03/Plots and display/Create Measurements [Pose]1/Create Measurements [Position]/Create Rotation Matrix /Create Skew Symmetric ==
  vector : Inport
  0 : Constant  Value=0
  Create 3x3 matrix : Subsystem
  Demux : Demux  Outputs=3
  Demux1 : Demux  Outputs=3
  Gain : Gain  Gain=-1
  skew symmetric Matrix : Outport
  wires:
  Demux1/1 -> Create 3x3 matrix/8(a32)
  Demux/2 -> Create 3x3 matrix/7(a31)
  Gain/1 -> Demux/1
  Create 3x3 matrix/1(Matrix) -> skew symmetric Matrix/1
  vector/1 -> Gain/1, Demux1/1
  Demux/1 -> Create 3x3 matrix/6(a23)
  Demux1/3 -> Create 3x3 matrix/4(a21)
  Demux1/2 -> Create 3x3 matrix/3(a13)
  Demux/3 -> Create 3x3 matrix/2(a12)
  0/1 -> Create 3x3 matrix/1(a11), Create 3x3 matrix/9(a33), Create 3x3 matrix/5(a22)

== system EKF_03/EKF/Measurement Update/Compute_K_d/Create H_k/Create Rotation Matrix /Create Skew Symmetric ==
  vector : Inport
  0 : Constant  Value=0
  Create 3x3 matrix : Subsystem
  Demux : Demux  Outputs=3
  Demux1 : Demux  Outputs=3
  Gain : Gain  Gain=-1
  skew symmetric Matrix : Outport
  wires:
  0/1 -> Create 3x3 matrix/1(a11), Create 3x3 matrix/9(a33), Create 3x3 matrix/5(a22)
  Demux/3 -> Create 3x3 matrix/2(a12)
  Demux1/2 -> Create 3x3 matrix/3(a13)
  Demux1/3 -> Create 3x3 matrix/4(a21)
  Demux/1 -> Create 3x3 matrix/6(a23)
  vector/1 -> Demux1/1, Gain/1
  Create 3x3 matrix/1(Matrix) -> skew symmetric Matrix/1
  Gain/1 -> Demux/1
  Demux/2 -> Create 3x3 matrix/7(a31)
  Demux1/1 -> Create 3x3 matrix/8(a32)

== system EKF_03/EKF/Measurement Update/Compute_K_d/Create H_k/Create Skew Symmetric/Create 3x3 matrix ==
  a11 : Inport
  a12 : Inport  Port=2
  a13 : Inport  Port=3
  a21 : Inport  Port=4
  a22 : Inport  Port=5
  a23 : Inport  Port=6
  a31 : Inport  Port=7
  a32 : Inport  Port=8
  a33 : Inport  Port=9
  Math Function : Math  Operator=transpose  SaturateOnIntegerOverflow=on
  Reshape (9) to [3x3] column-major : Reshape  OutputDimensionality=Customize  OutputDimensions=[3,3]
  Vector Concatenate : Concatenate  NumInputs=9
  Matrix : Outport
  wires:
  a33/1 -> Vector Concatenate/9
  a22/1 -> Vector Concatenate/5
  Vector Concatenate/1 -> Reshape (9) to [3x3] column-major/1
  a11/1 -> Vector Concatenate/1
  a12/1 -> Vector Concatenate/2
  a13/1 -> Vector Concatenate/3
  a23/1 -> Vector Concatenate/6
  a31/1 -> Vector Concatenate/7
  a32/1 -> Vector Concatenate/8
  a21/1 -> Vector Concatenate/4
  Reshape (9) to [3x3] column-major/1 -> Math Function/1
  Math Function/1 -> Matrix/1

== system EKF_03/EKF/Measurement Update/Create H_k/Create Rotation Matrix /Create Skew Symmetric/Create 3x3 matrix ==
  a11 : Inport
  a12 : Inport  Port=2
  a13 : Inport  Port=3
  a21 : Inport  Port=4
  a22 : Inport  Port=5
  a23 : Inport  Port=6
  a31 : Inport  Port=7
  a32 : Inport  Port=8
  a33 : Inport  Port=9
  Math Function : Math  Operator=transpose  SaturateOnIntegerOverflow=on
  Reshape (9) to [3x3] column-major : Reshape  OutputDimensionality=Customize  OutputDimensions=[3,3]
  Vector Concatenate : Concatenate  NumInputs=9
  Matrix : Outport
  wires:
  a33/1 -> Vector Concatenate/9
  a22/1 -> Vector Concatenate/5
  Vector Concatenate/1 -> Reshape (9) to [3x3] column-major/1
  a11/1 -> Vector Concatenate/1
  a12/1 -> Vector Concatenate/2
  a13/1 -> Vector Concatenate/3
  a23/1 -> Vector Concatenate/6
  a31/1 -> Vector Concatenate/7
  a32/1 -> Vector Concatenate/8
  a21/1 -> Vector Concatenate/4
  Reshape (9) to [3x3] column-major/1 -> Math Function/1
  Math Function/1 -> Matrix/1

== system EKF_03/EKF/Measurement Update/Create h/Create Rotation Matrix /Create Skew Symmetric/Create 3x3 matrix ==
  a11 : Inport
  a12 : Inport  Port=2
  a13 : Inport  Port=3
  a21 : Inport  Port=4
  a22 : Inport  Port=5
  a23 : Inport  Port=6
  a31 : Inport  Port=7
  a32 : Inport  Port=8
  a33 : Inport  Port=9
  Math Function : Math  Operator=transpose  SaturateOnIntegerOverflow=on
  Reshape (9) to [3x3] column-major : Reshape  OutputDimensionality=Customize  OutputDimensions=[3,3]
  Vector Concatenate : Concatenate  NumInputs=9
  Matrix : Outport
  wires:
  a33/1 -> Vector Concatenate/9
  a22/1 -> Vector Concatenate/5
  Vector Concatenate/1 -> Reshape (9) to [3x3] column-major/1
  a11/1 -> Vector Concatenate/1
  a12/1 -> Vector Concatenate/2
  a13/1 -> Vector Concatenate/3
  a23/1 -> Vector Concatenate/6
  a31/1 -> Vector Concatenate/7
  a32/1 -> Vector Concatenate/8
  a21/1 -> Vector Concatenate/4
  Reshape (9) to [3x3] column-major/1 -> Math Function/1
  Math Function/1 -> Matrix/1

== system EKF_03/EKF/Measurement Update/Create h_d/Create Rotation Matrix /Create Skew Symmetric/Create 3x3 matrix ==
  a11 : Inport
  a12 : Inport  Port=2
  a13 : Inport  Port=3
  a21 : Inport  Port=4
  a22 : Inport  Port=5
  a23 : Inport  Port=6
  a31 : Inport  Port=7
  a32 : Inport  Port=8
  a33 : Inport  Port=9
  Math Function : Math  Operator=transpose  SaturateOnIntegerOverflow=on
  Reshape (9) to [3x3] column-major : Reshape  OutputDimensionality=Customize  OutputDimensions=[3,3]
  Vector Concatenate : Concatenate  NumInputs=9
  Matrix : Outport
  wires:
  Math Function/1 -> Matrix/1
  Reshape (9) to [3x3] column-major/1 -> Math Function/1
  a21/1 -> Vector Concatenate/4
  a32/1 -> Vector Concatenate/8
  a31/1 -> Vector Concatenate/7
  a23/1 -> Vector Concatenate/6
  a13/1 -> Vector Concatenate/3
  a12/1 -> Vector Concatenate/2
  a11/1 -> Vector Concatenate/1
  Vector Concatenate/1 -> Reshape (9) to [3x3] column-major/1
  a22/1 -> Vector Concatenate/5
  a33/1 -> Vector Concatenate/9

== system EKF_03/EKF/Measurement Update/Propagate_state (full)/State Propagation1/Create M/Create 3x3 matrix ==
  a11 : Inport
  a12 : Inport  Port=2
  a13 : Inport  Port=3
  a21 : Inport  Port=4
  a22 : Inport  Port=5
  a23 : Inport  Port=6
  a31 : Inport  Port=7
  a32 : Inport  Port=8
  a33 : Inport  Port=9
  Math Function : Math  Operator=transpose  SaturateOnIntegerOverflow=on
  Reshape (9) to [3x3] column-major : Reshape  OutputDimensionality=Customize  OutputDimensions=[3,3]
  Vector Concatenate : Concatenate  NumInputs=9
  Matrix : Outport
  wires:
  a33/1 -> Vector Concatenate/9
  a22/1 -> Vector Concatenate/5
  Vector Concatenate/1 -> Reshape (9) to [3x3] column-major/1
  a11/1 -> Vector Concatenate/1
  a12/1 -> Vector Concatenate/2
  a13/1 -> Vector Concatenate/3
  a23/1 -> Vector Concatenate/6
  a31/1 -> Vector Concatenate/7
  a32/1 -> Vector Concatenate/8
  a21/1 -> Vector Concatenate/4
  Reshape (9) to [3x3] column-major/1 -> Math Function/1
  Math Function/1 -> Matrix/1

== system EKF_03/EKF/Predictor/Create State error covariance (P)/State Propagation/Create M/Create 3x3 matrix ==
  a11 : Inport
  a12 : Inport  Port=2
  a13 : Inport  Port=3
  a21 : Inport  Port=4
  a22 : Inport  Port=5
  a23 : Inport  Port=6
  a31 : Inport  Port=7
  a32 : Inport  Port=8
  a33 : Inport  Port=9
  Math Function : Math  Operator=transpose  SaturateOnIntegerOverflow=on
  Reshape (9) to [3x3] column-major : Reshape  OutputDimensionality=Customize  OutputDimensions=[3,3]
  Vector Concatenate : Concatenate  NumInputs=9
  Matrix : Outport
  wires:
  a33/1 -> Vector Concatenate/9
  a22/1 -> Vector Concatenate/5
  Vector Concatenate/1 -> Reshape (9) to [3x3] column-major/1
  a11/1 -> Vector Concatenate/1
  a12/1 -> Vector Concatenate/2
  a13/1 -> Vector Concatenate/3
  a23/1 -> Vector Concatenate/6
  a31/1 -> Vector Concatenate/7
  a32/1 -> Vector Concatenate/8
  a21/1 -> Vector Concatenate/4
  Reshape (9) to [3x3] column-major/1 -> Math Function/1
  Math Function/1 -> Matrix/1

== system EKF_03/EKF/Predictor/Dynamic Model (Differential equations)1/Dynamic Model (Differential equations)/Orbital Dynamics /Create Skew Symmetric ==
  vector : Inport
  0 : Constant  Value=0  SampleTime=-1
  Create 3x3 matrix : Subsystem
  Demux : Demux  Outputs=3
  Demux1 : Demux  Outputs=3
  Gain : Gain  Gain=-1
  skew symmetric Matrix : Outport
  wires:
  0/1 -> Create 3x3 matrix/9(a33), Create 3x3 matrix/5(a22), Create 3x3 matrix/1(a11)
  Demux/3 -> Create 3x3 matrix/2(a12)
  Demux1/2 -> Create 3x3 matrix/3(a13)
  Demux1/3 -> Create 3x3 matrix/4(a21)
  Demux/1 -> Create 3x3 matrix/6(a23)
  vector/1 -> Demux1/1, Gain/1
  Create 3x3 matrix/1(Matrix) -> skew symmetric Matrix/1
  Gain/1 -> Demux/1
  Demux/2 -> Create 3x3 matrix/7(a31)
  Demux1/1 -> Create 3x3 matrix/8(a32)

== system EKF_03/EKF/Predictor/Dynamic Model (Differential equations)1/Dynamic Model (Differential equations)/Orbital Dynamics /norm  ==
  vector : Inport
  Dot Product : DotProduct  InputSameDT=on  OutDataTypeStr=Inherit: Inherit via internal rule
  Sqrt : Sqrt  SaturateOnIntegerOverflow=on
  "norm " : Outport
  wires:
  Dot Product/1 -> Sqrt/1
  vector/1 -> Dot Product/2, Dot Product/1
  Sqrt/1 -> "norm "/1

== system EKF_03/EKF/Predictor/Dynamic Model (Differential equations)1/Dynamic Model (Differential equations)/Rotational Dynamics/Create  J ==
  p : Inport
  0 : Constant  Value=0  SampleTime=-1
  1 : Constant  SampleTime=-1
  Create 3x3 matrix : Subsystem
  Fcn : Fcn  Expr=1-u(2)/1+u(1)
  Fcn1 : Fcn  Expr=1+u(3)/1-u(1)
  "J_k " : Outport
  wires:
  Fcn/1 -> Create 3x3 matrix/5(a22)
  p/1 -> Fcn1/1, Fcn/1
  0/1 -> Create 3x3 matrix/8(a32), Create 3x3 matrix/7(a31), Create 3x3 matrix/6(a23), Create 3x3 matrix/4(a21), Create 3x3 matrix/3(a13), Create 3x3 matrix/2(a12)
  Create 3x3 matrix/1(Matrix) -> "J_k "/1
  Fcn1/1 -> Create 3x3 matrix/9(a33)
  1/1 -> Create 3x3 matrix/1(a11)

== system EKF_03/EKF/Predictor/Dynamic Model (Differential equations)1/Dynamic Model (Differential equations)/Rotational Dynamics/Create Psi ==
  "omega " : Inport
  p : Inport  Port=2
  Create Psi : Concatenate  NumInputs=3
  Demux : Demux  Outputs=3
  Demux1 : Demux  Outputs=3
  Product{,1..5} (6 alike) : Product
  Scope : Scope
      settings: SaveName=ScopeData20
  Psi : Outport
  wires:
  Demux1/3 -> Product1/2, Product3/2
  p/1 -> Demux/1
  Demux/3 -> Product4/1
  Product4/1 -> Create Psi/3
  Demux1/1 -> Product5/2, Product3/1
  Demux1/2 -> Product1/1, Product5/1
  Product2/1 -> Create Psi/2
  Demux/1 -> Product/1
  Create Psi/1 -> Scope/1, Psi/1
  Demux/2 -> Product2/1
  Product/1 -> Create Psi/1
  Product1/1 -> Product/2
  Product5/1 -> Product4/2
  Product3/1 -> Product2/2
  "omega "/1 -> Demux1/1
